simulink model "controller2_SR"  (R2025b)
settings: Solver=VariableStepAuto  StartTime=0.0  StopTime=10.0  RelTol=1e-3
values from neighbouring files (symbols this model uses):
  A = [0 1; -k/J -b/J]    [sofia_udp_test.m]
  b = 0.05    [sofia_udp_test.m]
  B = [0; 1/J]    [sofia_udp_test.m]
  C = [1 0]    [sofia_udp_test.m]
  D = zeros()    [sofia_udp_test.m]
  k = 0.1    [sofia_udp_test.m]
  omega_c = 62    [sofia_udp_test.m]
  Ts = mean(valid_dt)    [capt_est_params.m]    (also in capt_fidel_castro.m = mean(diff(time_data)); capt_id.m = mean(diff(time_data)); for_mat.m = mean(diff(seg_time)); sofia_udp_test.m = 0.001)
undefined symbols (not defined in the file or in its folder): den_d, num_d
libraries: etargetslib x1, instrumentlib x1
settings Model: Creator=javot  LastModifiedBy=sofia
settings SolverCC: AlgebraicLoopSolver=TrustRegion
settings DebuggingCC: UnconnectedInputMsg=warning  UnconnectedOutputMsg=warning  UnconnectedLineMsg=warning
settings ModelReferenceCC: EnableRefExpFcnMdlSchedulingChecks=on
settings RTWCC: GPUComputeCapability=3.5

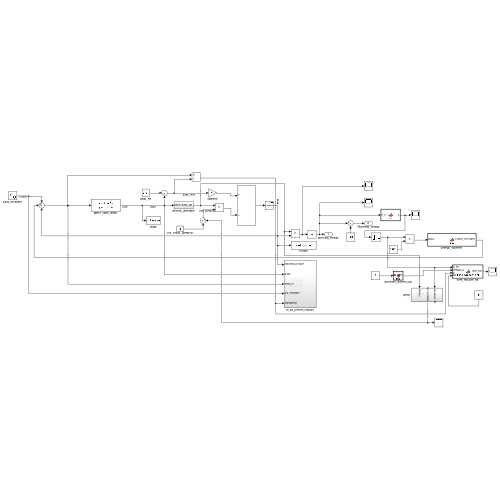
[thumbnail: Simulink's stored preview of the top-level diagram]
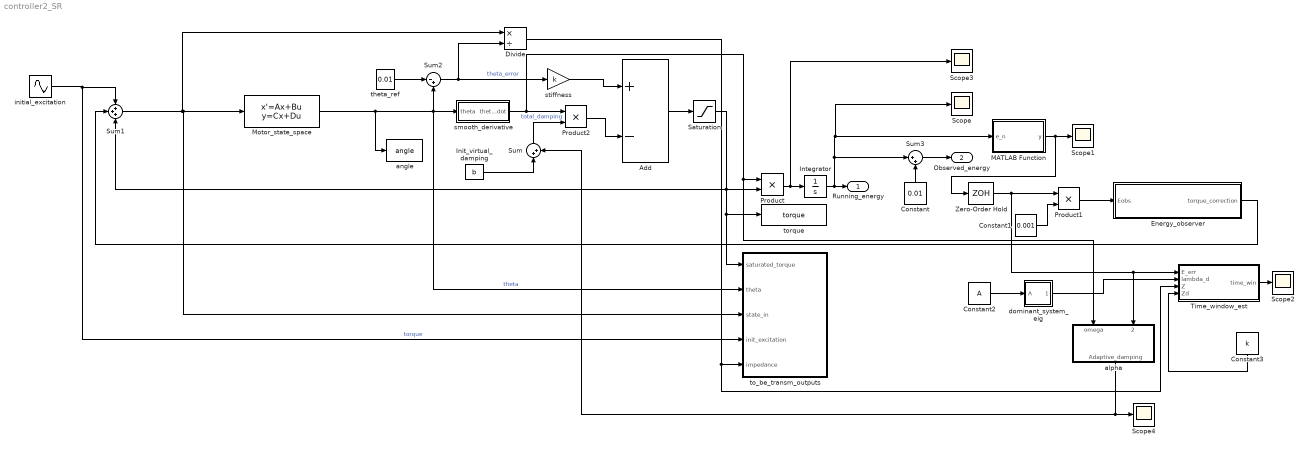
== system controller2_SR ==
  Add : Sum  Inputs=+-
  Constant : Constant  Value=0.01
  Constant1 : Constant  Value=0.001
  Constant2 : Constant  Value=A
  Constant3 : Constant  Value=k
  Divide : Product  Inputs=*/
  Energy_observer : MATLAB Function  TreatAsAtomicUnit=on
  Init_virtual_damping : Constant  Value=b
  Integrator : Integrator  InitialCondition=0.01
  MATLAB Function : MATLAB Function  TreatAsAtomicUnit=on
  Motor_state_space : StateSpace  A=A  B=B  C=C  D=D  InitialCondition=0  ContinuousStateAttributes="\"\""
  Product : Product
  Product1 : Product
  Product2 : Product
  Saturation : Saturate  UpperLimit=1  LowerLimit=-1
  Scope{,1..4} (5 alike) : Scope
      Scope settings: ActiveDisplayYMinimum=-1  ActiveDisplayYMaximum=1
      Scope1 settings: ActiveDisplayYMinimum=-0.012016913140581283  ActiveDisplayYMaximum=0.010705981782451628  DataLoggingVariableName=ScopeData2
      Scope2 settings: ActiveDisplayYMinimum=0.155737570978111  ActiveDisplayYMaximum=0.53497513283526754
      Scope3 settings: ActiveDisplayYMinimum=-1  ActiveDisplayYMaximum=1  DataLoggingVariableName=ScopeData3
      Scope4 settings: ActiveDisplayYMinimum=0.00051322743836190276  ActiveDisplayYMaximum=0.00099244253542332531  DataLoggingVariableName=ScopeData4
  Sum : Sum  Inputs=|++
  Sum1 : Sum  Inputs=+++
  Sum2 : Sum  Inputs=|-+
  Sum3 : Sum  Inputs=|++
  Time_window_est : MATLAB Function  TreatAsAtomicUnit=on
  Zero-Order Hold : ZeroOrderHold  SampleTime=Ts
  alpha : Subsystem
  angle : ToWorkspace  VariableName=angle  SaveFormat=Timeseries  SampleTime=-1
  dominant_system_eig : MATLAB Function  TreatAsAtomicUnit=on
  initial_excitation : Sin  SampleTime=Ts
  smooth_derivative : Subsystem
  stiffness : Gain  Gain=k
  theta_ref : Constant  Value=0.01
  to_be_transm_outputs : Subsystem
  torque : ToWorkspace  VariableName=torque  SaveFormat=Timeseries  SampleTime=-1
  Running_energy : Outport
  Observed_energy : Outport  Port=2
  wires:
  Sum2/1 -> stiffness/1, Divide/2  "theta_error"
  Sum1/1 -> to_be_transm_outputs/3(state_in), Motor_state_space/1, Divide/1
  Add/1 -> Saturation/1
  MATLAB Function/1(y) -> Zero-Order Hold/1, Scope1/1
  stiffness/1 -> Add/1
  Sum3/1 -> Observed_energy/1
  initial_excitation/1 -> to_be_transm_outputs/4(init_excitation), Sum1/1  "torque"
  Constant/1 -> Sum3/2
  Divide/1 -> to_be_transm_outputs/5(impedance), Time_window_est/3(Z)
  Motor_state_space/1 -> to_be_transm_outputs/2(theta), Sum2/2, smooth_derivative/1(theta), angle/1  "theta"
  Saturation/1 -> Sum1/3, Product/2, torque/1, to_be_transm_outputs/1(saturated_torque)
  Product2/1 -> Add/2
  theta_ref/1 -> Sum2/1
  smooth_derivative/1(theta_dot) -> alpha/1(omega), Product/1, Product2/1
  Product/1 -> Integrator/1, Scope3/1
  Zero-Order Hold/1 -> Time_window_est/1(E_err), alpha/2(Energy_observed), Product1/1
  Constant1/1 -> Product1/2
  Product1/1 -> Energy_observer/1(Eobs)
  Energy_observer/1(torque_correction) -> Sum1/2
  Init_virtual_damping/1 -> Sum/1
  Sum/1 -> Product2/2  "total_damping"
  dominant_system_eig/1(lambda_dom) -> Time_window_est/2(lambda_d)
  Constant2/1 -> dominant_system_eig/1(A)
  Constant3/1 -> Time_window_est/4(Zd)
  Time_window_est/1(time_win) -> Scope2/1
  alpha/1(Adaptive_damping) -> Sum/2, Scope4/1
  Integrator/1 -> Scope/1, MATLAB Function/1(e_n), Sum3/1, Running_energy/1

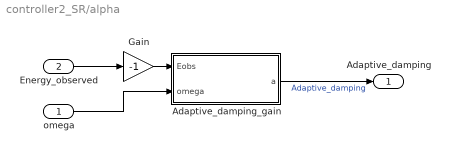
== system controller2_SR/alpha ==
  omega : Inport
  Energy_observed : Inport  Port=2
  Adaptive_damping_gain : MATLAB Function  TreatAsAtomicUnit=on
  Gain : Gain  Gain=-1
  Adaptive_damping : Outport
  wires:
  Energy_observed/1 -> Gain/1
  Gain/1 -> Adaptive_damping_gain/1(Eobs)
  Adaptive_damping_gain/1(a) -> Adaptive_damping/1  "Adaptive_damping"
  omega/1 -> Adaptive_damping_gain/2(omega)

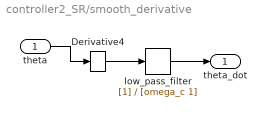
== system controller2_SR/smooth_derivative ==
  theta : Inport
  Derivative4 : Derivative
  low_pass_filter : TransferFcn  Denominator=[omega_c 1]
  theta_dot : Outport
  wires:
  Derivative4/1 -> low_pass_filter/1
  theta/1 -> Derivative4/1
  low_pass_filter/1 -> theta_dot/1

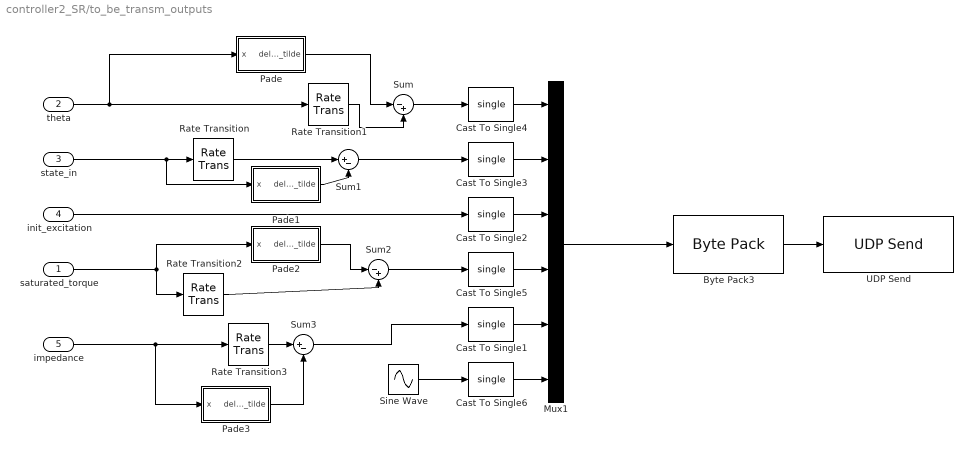
== system controller2_SR/to_be_transm_outputs ==
  saturated_torque : Inport
  theta : Inport  Port=2
  state_in : Inport  Port=3
  init_excitation : Inport  Port=4
  impedance : Inport  Port=5
  Byte Pack3 : etargetslib/Byte Pack  datatypes={'single'}  byteAlign=1
  Cast To Single{1..6} (6 alike) : DataTypeConversion  OutDataTypeStr=single  SaturateOnIntegerOverflow=off  RndMeth=Floor
  Mux1 : Mux  Inputs=6
  Pade : Subsystem
  Pade1 : Subsystem
  Pade2 : Subsystem
  Pade3 : Subsystem
  Rate Transition{,1..3} (4 alike) : RateTransition
  Sine Wave : Sin  SampleTime=0.001
  Sum : Sum  Inputs=|-+
  Sum1 : Sum  Inputs=|+-
  Sum2 : Sum  Inputs=|-+
  Sum3 : Sum  Inputs=|+-
  UDP Send : instrumentlib/UDP Send  Host=134.105.60.99  Port=55001  LocalAddress=0.0.0.0  LocalPort=-1  EnablePortSharing=off  OutputDatagramPacketSize=512  ByteOrder=big-endian  EnableBlockingMode=on  SimulateUsing=Interpreted execution
  wires:
  Byte Pack3/1 -> UDP Send/1
  Mux1/1 -> Byte Pack3/1
  Sine Wave/1 -> Cast To Single6/1
  init_excitation/1 -> Cast To Single2/1
  theta/1 -> Pade/1(x), Rate Transition1/1
  saturated_torque/1 -> Pade2/1(x), Rate Transition2/1
  impedance/1 -> Pade3/1(x), Rate Transition3/1
  Cast To Single4/1 -> Mux1/1
  Cast To Single3/1 -> Mux1/2
  Cast To Single5/1 -> Mux1/4
  Cast To Single2/1 -> Mux1/3
  Cast To Single1/1 -> Mux1/5
  Cast To Single6/1 -> Mux1/6
  Rate Transition1/1 -> Sum/2
  Sum/1 -> Cast To Single4/1
  Rate Transition/1 -> Sum1/1
  Sum1/1 -> Cast To Single3/1
  Rate Transition2/1 -> Sum2/2
  Sum2/1 -> Cast To Single5/1
  Rate Transition3/1 -> Sum3/1
  Sum3/1 -> Cast To Single1/1
  state_in/1 -> Pade1/1(x), Rate Transition/1
  Pade2/1(delay_tilde) -> Sum2/1
  Pade/1(delay_tilde) -> Sum/1
  Pade1/1(delay_tilde) -> Sum1/2
  Pade3/1(delay_tilde) -> Sum3/2

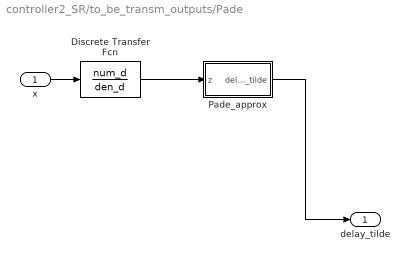
== system controller2_SR/to_be_transm_outputs/Pade ==
  x : Inport
  Discrete Transfer Fcn : DiscreteTransferFcn  Numerator=num_d  Denominator=den_d
  Pade_approx : MATLAB Function  TreatAsAtomicUnit=on
  delay_tilde : Outport
  wires:
  Discrete Transfer Fcn/1 -> Pade_approx/1(z)
  Pade_approx/1(delay_tilde) -> delay_tilde/1
  x/1 -> Discrete Transfer Fcn/1

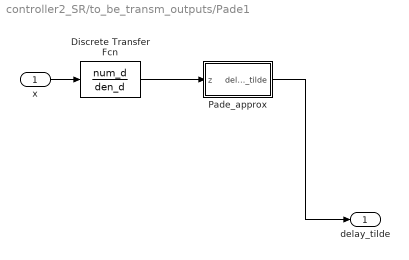
== system controller2_SR/to_be_transm_outputs/Pade1 ==
  x : Inport
  Discrete Transfer Fcn : DiscreteTransferFcn  Numerator=num_d  Denominator=den_d
  Pade_approx : MATLAB Function  TreatAsAtomicUnit=on
  delay_tilde : Outport
  wires:
  Discrete Transfer Fcn/1 -> Pade_approx/1(z)
  Pade_approx/1(delay_tilde) -> delay_tilde/1
  x/1 -> Discrete Transfer Fcn/1

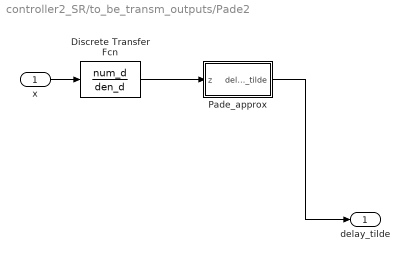
== system controller2_SR/to_be_transm_outputs/Pade2 ==
  x : Inport
  Discrete Transfer Fcn : DiscreteTransferFcn  Numerator=num_d  Denominator=den_d
  Pade_approx : MATLAB Function  TreatAsAtomicUnit=on
  delay_tilde : Outport
  wires:
  Discrete Transfer Fcn/1 -> Pade_approx/1(z)
  Pade_approx/1(delay_tilde) -> delay_tilde/1
  x/1 -> Discrete Transfer Fcn/1

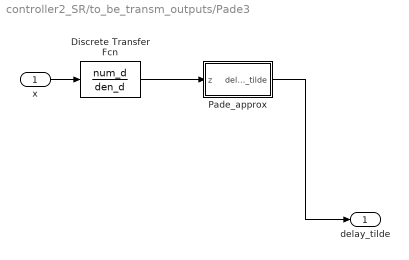
== system controller2_SR/to_be_transm_outputs/Pade3 ==
  x : Inport
  Discrete Transfer Fcn : DiscreteTransferFcn  Numerator=num_d  Denominator=den_d
  Pade_approx : MATLAB Function  TreatAsAtomicUnit=on
  delay_tilde : Outport
  wires:
  Discrete Transfer Fcn/1 -> Pade_approx/1(z)
  Pade_approx/1(delay_tilde) -> delay_tilde/1
  x/1 -> Discrete Transfer Fcn/1

== matlab function controller2_SR/to_be_transm_outputs/Pade1/Pade_approx ==
  data: delay_tilde output; z input
function delay_tilde= fcn(z)
persistent z_prev; 
persistent delay_prev;

if isempty(z_prev)
    z_prev = 0;
    delay_prev = 0;
end
delay_tilde = z/3 + z_prev + (1/3)*delay_prev;
z_prev = z;
delay_prev = delay_tilde;

end

== matlab function controller2_SR/to_be_transm_outputs/Pade/Pade_approx ==
  data: delay_tilde output; z input
function delay_tilde= fcn(z)
persistent z_prev; 
persistent delay_prev;

if isempty(z_prev)
    z_prev = 0;
    delay_prev = 0;
end
delay_tilde = z/3 + z_prev + (1/3)*delay_prev;
z_prev = z;
delay_prev = delay_tilde;

end

== matlab function controller2_SR/to_be_transm_outputs/Pade2/Pade_approx ==
  data: delay_tilde output; z input
function delay_tilde= fcn(z)
persistent z_prev; 
persistent delay_prev;

if isempty(z_prev)
    z_prev = 0;
    delay_prev = 0;
end
delay_tilde = z/3 + z_prev + (1/3)*delay_prev;
z_prev = z;
delay_prev = delay_tilde;

end

== matlab function controller2_SR/to_be_transm_outputs/Pade3/Pade_approx ==
  data: delay_tilde output; z input
function delay_tilde= fcn(z)
persistent z_prev; 
persistent delay_prev;

if isempty(z_prev)
    z_prev = 0;
    delay_prev = 0;
end
delay_tilde = z/3 + z_prev + (1/3)*delay_prev;
z_prev = z;
delay_prev = delay_tilde;

end

== matlab function controller2_SR/MATLAB Function ==
  settings: updateMethod=DISCRETE
  data: e_n input; y output
function y = fcn(e_n)

persistent e_prev

if isempty(e_prev)
    e_prev = 0.01;      % initial condition
end

y = e_n - e_prev;

e_prev = y;

== matlab function controller2_SR/Energy_observer ==
  data: Eobs input; torque_correction output
function torque_correction = fcn(Eobs)

torque_correction = Eobs;

== matlab function controller2_SR/alpha/Adaptive_damping_gain ==
  settings: updateMethod=DISCRETE
  data: Eobs input; a output; omega input
function a = fcn(Eobs, omega)

persistent a_prev

% Parameters
deltaT = 0.001;
omega_min = 1e-3;     % Prevent division by zero
a_min = 0.001;
a_max = 100;          % Adjust according to your application

% Initialization
if isempty(a_prev)
    a_prev = 1e-4;
end

% Safe angular velocity
omega_safe = max(abs(omega), omega_min);

% Adaptation law
if Eobs < 0
    a = a_prev + Eobs/(deltaT*omega_safe^2);
else
    % Keep previous value instead of resetting
    a = a_prev;
end

% Saturation
a = min(max(a, a_min), a_max);

% Store for next iteration
a_prev = a;

end

== matlab function controller2_SR/Time_window_est ==
  settings: updateMethod=DISCRETE
  data: E_err input; time_win output; lambda_d input; Z input; Zd input
function time_win = Time_window_est(E_err, lambda_d, Z, Zd)
%#codegen
%
% Estimates an adaptive observation window using:
%   1. dominant closed-loop eigenvalue,
%   2. normalized energy error,
%   3. normalized impedance error,
%   4. zero-crossing-rate history of the energy-error signal.
%
% Inputs:
%   E_err     - instantaneous energy/transparency error [J]
%   lambda_d  - dominant closed-loop eigenvalue
%   Z         - measured impedance, scalar or fixed-size vector
%   Zd        - desired impedance, scalar or fixed-size vector
%
% Output:
%   time_win  - estimated time window [s]

persistent E_history
persistent history_index
persistent sample_count
persistent zcr_filtered
persistent t_prev

%% Parameters
Tmin = 0.01;             % Minimum window: 10 ms
Tmax = 0.50;             % Maximum window: 500 ms

Eref = 1e-3;             % Reference energy [J]
tau_min = 1e-3;          % Minimum characteristic time [s]
tau_max = 0.50;          % Maximum characteristic time [s]

history_length = 100;    % Number of stored E_err samples

alpha_zcr = 0.10;        % ZCR low-pass filtering factor
alpha_time = 0.10;       % Window low-pass filtering factor

k_energy = 1.0;          % Energy-error contribution
k_impedance = 1.0;       % Impedance-error contribution
k_zcr = 2.0;             % ZCR contribution

zero_threshold = 1e-9;   % Prevent noise around zero from causing crossings

%% Initialization
if isempty(E_history)
    E_history = zeros(history_length, 1);
    history_index = 1;
    sample_count = 0;
    zcr_filtered = 0;
    t_prev = 0.05;       % Initial window: 50 ms
end

%% Store current energy-error sample
E_history(history_index) = E_err;

history_index = history_index + 1;

if history_index > history_length
    history_index = 1;
end

if sample_count < history_length
    sample_count = sample_count + 1;
end

%% Compute zero-crossing rate from available history
zero_crossings = 0;

if sample_count >= 2

    % Reconstruct the history in chronological order.
    ordered_history = zeros(history_length, 1);

    if sample_count < history_length
        ordered_history(1:sample_count) = E_history(1:sample_count);
    else
        output_index = 1;

        for input_index = history_index:history_length
            ordered_history(output_index) = E_history(input_index);
            output_index = output_index + 1;
        end

        for input_index = 1:(history_index - 1)
            ordered_history(output_index) = E_history(input_index);
            output_index = output_index + 1;
        end
    end

    % Count sign changes while ignoring very small values.
    for i = 2:sample_count

        previous_value = ordered_history(i - 1);
        current_value = ordered_history(i);

        previous_is_positive = previous_value > zero_threshold;
        previous_is_negative = previous_value < -zero_threshold;

        current_is_positive = current_value > zero_threshold;
        current_is_negative = current_value < -zero_threshold;

        crossed_zero = ...
            (previous_is_positive && current_is_negative) || ...
            (previous_is_negative && current_is_positive);

        if crossed_zero
            zero_crossings = zero_crossings + 1;
        end
    end

    % Normalized ZCR in the interval [0,1].
    zcr_current = zero_crossings / (sample_count - 1);

else
    zcr_current = 0;
end

%% Smooth the ZCR estimate
zcr_filtered = ...
    (1 - alpha_zcr) * zcr_filtered + ...
    alpha_zcr * zcr_current;

%% Characteristic system time from dominant eigenvalue
lambda_real = real(lambda_d);

if lambda_real < -1e-9
    tau_c = -1 / lambda_real;
else
    % Unstable or nearly marginal eigenvalue.
    % Select the largest permitted characteristic time.
    tau_c = tau_max;
end

tau_c = min(max(tau_c, tau_min), tau_max);

%% Normalized impedance error
Zd_norm = norm(Zd);

if Zd_norm < 1e-12
    Zd_norm = 1e-12;
end

impedance_error = norm(Z - Zd) / Zd_norm;

%% Normalized energy error
energy_error = abs(E_err) / max(Eref, 1e-12);

%% Limit normalized errors to prevent extreme window commands
energy_error = min(energy_error, 10);
impedance_error = min(impedance_error, 10);

%% Adaptive candidate window
%
% Larger energy or impedance error increases the observation window.
% Larger ZCR decreases it so that the controller responds more quickly
% to rapidly changing interaction dynamics.

time_candidate = tau_c * ...
    (1 + k_energy * energy_error + ...
         k_impedance * impedance_error) / ...
    (1 + k_zcr * zcr_filtered);

%% Saturate candidate window
time_candidate = min(max(time_candidate, Tmin), Tmax);

%% Smooth the time-window command
time_win = ...
    (1 - alpha_time) * t_prev + ...
    alpha_time * time_candidate;

%% Final saturation and state update
time_win = min(max(time_win, Tmin), Tmax);

t_prev = time_win;

end

== matlab function controller2_SR/dominant_system_eig ==
  data: A input; lambda_dom output
function lambda_dom = fcn(A)

lambdas = eig(A);
[~,idx] = max(real(lambdas));
lambda_dom = lambdas(idx);
